simulink model "SeriesConnection"  (R2024a)
settings: Solver=VariableStepAuto  StartTime=0.0  StopTime=10.0  RelTol=1e-3
libraries: cstblocks x4
settings Model: Creator=PMYLS  LastModifiedBy=PMYLS

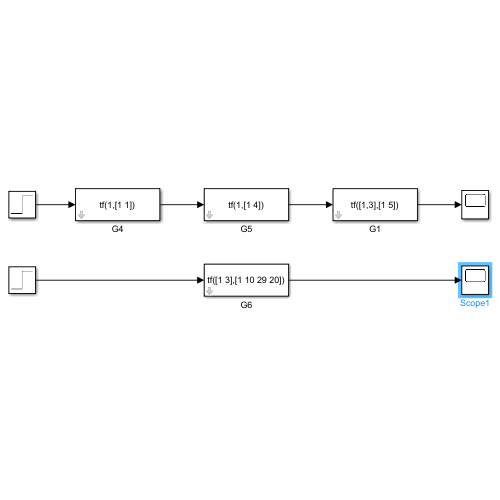
[thumbnail: Simulink's stored preview of the top-level diagram]
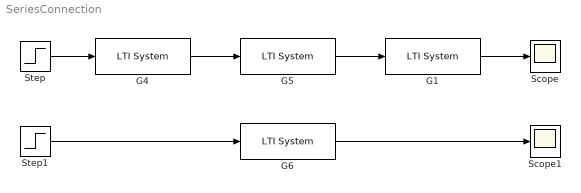
== system SeriesConnection ==
  G1 : cstblocks/LTI System  sys=tf([1,3],[1 5])  IC=[]  PadeOrder=0
  G4 : cstblocks/LTI System  sys=tf(1,[1 1])  IC=[]  PadeOrder=0
  G5 : cstblocks/LTI System  sys=tf(1,[1 4])  IC=[]  PadeOrder=0
  G6 : cstblocks/LTI System  sys=tf([1 3],[1 10 29 20])  IC=[]  PadeOrder=0
  Scope : Scope
  Scope1 : Scope
  Step : Step  SampleTime=0
  Step1 : Step  SampleTime=0
  wires:
  G4/1 -> G5/1
  G5/1 -> G1/1
  Step/1 -> G4/1
  G1/1 -> Scope/1
  G6/1 -> Scope1/1
  Step1/1 -> G6/1
